simulink model "Sim_Ex25"  (R2017a)
settings: Solver=ode45  StartTime=0  StopTime=Stop_Time  MaxStep=Ts  RelTol=1e-3  EnableMultiTasking=on
values from neighbouring files (symbols this model uses):
  Lamf = 0.254    [A_Ex25.m]
  Lamf_Hat = 1.0*Lamf    (= 0.254)    [A_Ex25.m]
  Lds = 3.6e-3    (= 0.0036)    [A_Ex25.m]
  Lds_Hat = 1.0*Lds    (= 0.0036)    [A_Ex25.m]
  Lqs = 4.3e-3    (= 0.0043)    [A_Ex25.m]
  Lqs_Hat = 1.0*Lqs    (= 0.0043)    [A_Ex25.m]
  p = 3    [A_Ex25.m]
  Rs = 0.15    [A_Ex25.m]
  Step_Time = 0.05    [A_Ex25.m]
  Stop_Time = 0.25    [A_Ex25.m]
  Te_Rated = interp1(MTPA.Is(Ind_PosTe),MTPA.Te(Ind_PosTe),Is_Rated)    [A_Ex25.m]
  Te_Ref_Set = [0 1]*Te_Rated    [A_Ex25.m]
  Te_SlewRate = 10    [A_Ex25.m]
  Thetarm_Init = 0*pi*1/p    (= 0)    [A_Ex25.m]
  Ts = 1/fs    (= 5e-05)    [A_Ex25.m]
  Tsw = 1/fsw    (= 0.0001)    [A_Ex25.m]
  Vdc = 310    [A_Ex25.m]
  Wrm_Fin = 2000*2*pi/60    (= 209.439510239)    [A_Ex25.m]
  Wrm_Init = 2000*2*pi/60    (= 209.439510239)    [A_Ex25.m]
undefined symbols (not defined in the file or in its folder): CC, DiscIntNeverNeededParam, FW, Mode, MTPA
libraries: simulink x7
settings Model: SimulationMode=accelerator  Creator=KYC  LastModifiedBy=KYC
settings DataIOCC: LimitDataPoints=on  SaveFormat=Array
settings OptimizationCC: LifeSpan=inf
settings DebuggingCC: UnderspecifiedInitializationDetection=Classic  MergeDetectMultiDrivingBlocksExec=none  SolverPrmCheckMsg=warning  InheritedTsInSrcMsg=none  AllowSymbolicDim=off  StateNameClashWarn=warning  SFUnexpectedBacktrackingDiag=warning  SFNoUnconditionalDefaultTransitionDiag=warning  SFExecutionAtInitializationDiag=none
settings HardwareCC: ProdBitPerPointer=32  ProdBitPerSizeT=32  ProdBitPerPtrDiffT=32  ProdLargestAtomicFloat=None  ProdIntDivRoundTo=Undefined  ProdEndianess=Unspecified  ProdWordSize=32  ProdHWDeviceType=32-bit Generic
settings ModelReferenceCC: PropagateSignalLabelsOutOfModel=off
settings GRTTargetCC: TargetLangStandard=C89/C90 (ANSI)  GeneratePreprocessorConditionals=Disable all
settings ConfigComp: CovMetricSettings=dw  CovHtmlReporting=on  CovSaveCumulativeToWorkspaceVar=on  CovSaveSingleToWorkspaceVar=on  CovExternalEMLEnable=off  CovSFcnEnable=off

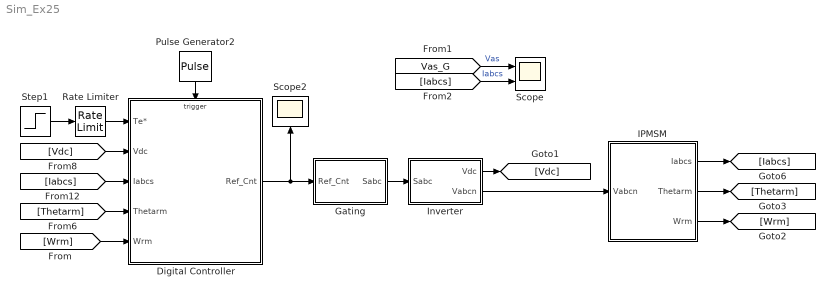
== system Sim_Ex25 ==
  Digital Controller : Subsystem
  Gating : Subsystem
  IPMSM : Subsystem
  Inverter : Subsystem
  Pulse Generator2 : DiscretePulseGenerator  PulseType=Time based  Period=Ts  PulseWidth=50
  Rate Limiter : RateLimiter  RisingSlewLimit=Te_SlewRate*Te_Rated  FallingSlewLimit=-Te_SlewRate*Te_Rated  SampleTimeMode=inherited
  Scope : Scope  NumInputPorts=2
  Scope2 : Scope
  Step1 : Step  Time=Step_Time  Before=Te_Ref_Set(:,1)  After=Te_Ref_Set(:,2)
  wires:
  Pulse Generator2/1 -> Digital Controller/Trigger
  [Vdc] -> Digital Controller/2(Vdc)
  Digital Controller/1(Ref_Cnt) -> Gating/1(Ref_Cnt), Scope2/1
  [Thetarm] -> Digital Controller/4(Thetarm)
  Gating/1(Sabc) -> Inverter/1(Sabc)
  [Iabcs] -> Digital Controller/3(Iabcs)
  Inverter/2(Vabcn) -> IPMSM/1(Vabcn)
  Inverter/1(Vdc) -> [Vdc]
  [Vas_G] -> Scope/1  "Vas"
  [Iabcs] -> Scope/2  "Iabcs"
  IPMSM/1(Iabcs) -> [Iabcs]
  IPMSM/2(Thetarm) -> [Thetarm]
  IPMSM/3(Wrm) -> [Wrm]
  Rate Limiter/1 -> Digital Controller/1(Te*)
  [Wrm] -> Digital Controller/5(Wrm)
  Step1/1 -> Rate Limiter/1

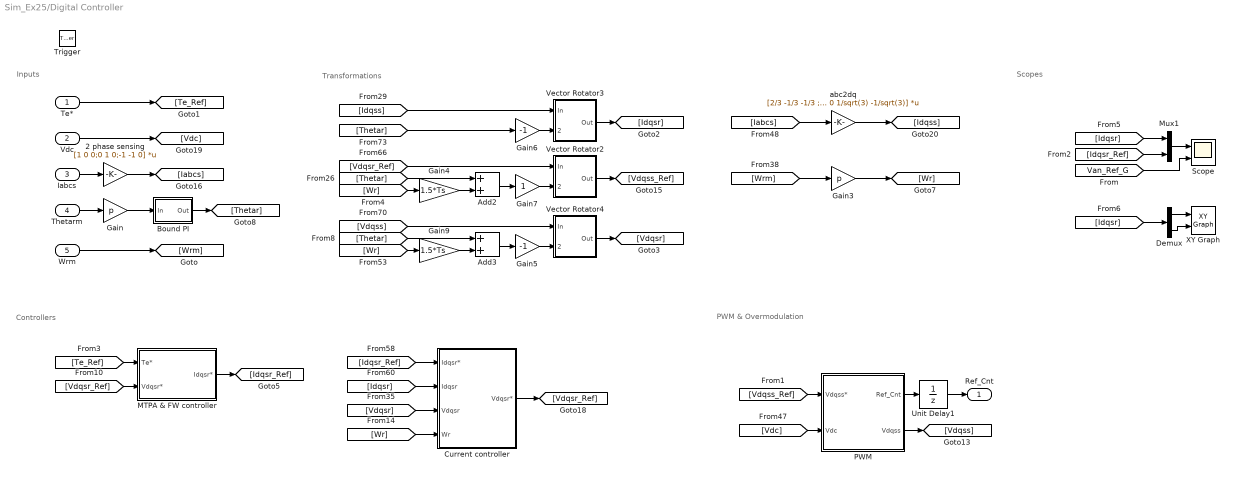
== system Sim_Ex25/Digital Controller ==
  note: PWM & Overmodulation
  note: Controllers
  note: Inputs
  note: Transformations
  note: Scopes
  Te* : Inport
  Vdc : Inport  Port=2
  Iabcs : Inport  Port=3
  Thetarm : Inport  Port=4
  Wrm : Inport  Port=5
  Trigger : TriggerPort  VariantControl=Variant
  2 phase sensing : Gain  Gain=[1 0 0;0 1 0;-1 -1 0]  Multiplication=Matrix(K*u)  SaturateOnIntegerOverflow=on  OutDataTypeStr=Inherit: Same as input  ParamDataTypeStr=Inherit: Same as input
  Add2 : Sum
  Add3 : Sum
  Bound PI : Subsystem
  Current controller : Subsystem
  Demux : Demux  Outputs=2
  Gain : Gain  Gain=p
  Gain3 : Gain  Gain=p
  Gain4 : Gain  Gain=1.5*Ts
  Gain5 : Gain  Gain=-1
  Gain6 : Gain  Gain=-1
  Gain7 : Gain
  Gain9 : Gain  Gain=1.5*Ts
  MTPA & FW controller : Subsystem
  Mux1 : Mux  Inputs=2
  PWM : Subsystem
  Scope : Scope  NumInputPorts=2
  Unit Delay1 : UnitDelay  SampleTime=-1
  Vector Rotator2 : Subsystem
  Vector Rotator3 : Subsystem
  Vector Rotator4 : Subsystem
  XY Graph : simulink/Sinks/XY Graph  xmin=-60  xmax=0  ymin=0  ymax=60  st=-1
  abc2dq : Gain  Gain=[2/3 -1/3 -1/3 ; 0 1/sqrt(3) -1/sqrt(3)]  Multiplication=Matrix(K*u)  SaturateOnIntegerOverflow=on  OutDataTypeStr=Inherit: Same as input  ParamDataTypeStr=Inherit: Same as input
  Ref_Cnt : Outport  InitialOutput=[0]
  wires:
  [Idqsr] -> Current controller/2(Idqsr)
  abc2dq/1 -> [Idqss]
  [Iabcs] -> abc2dq/1
  Vdc/1 -> [Vdc]
  [Vdqsr] -> Current controller/3(Vdqsr)
  [Idqsr_Ref] -> Current controller/1(Idqsr*)
  Thetarm/1 -> Gain/1
  [Wr] -> Current controller/4(Wr)
  Gain/1 -> Bound PI/1(In)
  Bound PI/1(Out) -> [Thetar]
  Current controller/1(Vdqsr*) -> [Vdqsr_Ref]
  Unit Delay1/1 -> Ref_Cnt/1
  PWM/2(Vdqss) -> [Vdqss]
  [Vdc] -> PWM/2(Vdc)
  Add2/1 -> Gain7/1
  Gain7/1 -> Vector Rotator2/2(Theta)
  [Vdqsr_Ref] -> Vector Rotator2/1(In)
  Vector Rotator2/1(Out) -> [Vdqss_Ref]
  [Wr] -> Gain9/1
  Gain9/1 -> Add3/2
  Add3/1 -> Gain5/1
  [Thetar] -> Add3/1
  Gain5/1 -> Vector Rotator4/2(Theta)
  [Vdqss] -> Vector Rotator4/1(In)
  Vector Rotator4/1(Out) -> [Vdqsr]
  [Vdqss_Ref] -> PWM/1(Vdqss*)
  Gain6/1 -> Vector Rotator3/2(Theta)
  [Idqss] -> Vector Rotator3/1(In)
  Vector Rotator3/1(Out) -> [Idqsr]
  [Thetar] -> Gain6/1
  PWM/1(Ref_Cnt) -> Unit Delay1/1
  Iabcs/1 -> 2 phase sensing/1
  2 phase sensing/1 -> [Iabcs]
  [Wr] -> Gain4/1
  Gain4/1 -> Add2/2
  [Thetar] -> Add2/1
  [Van_Ref_G] -> Scope/2
  Te*/1 -> [Te_Ref]
  [Idqsr] -> Demux/1
  Demux/2 -> XY Graph/2
  Demux/1 -> XY Graph/1
  [Idqsr_Ref] -> Mux1/2
  Mux1/1 -> Scope/1
  [Idqsr] -> Mux1/1
  [Vdqsr_Ref] -> MTPA & FW controller/2(Vdqsr*)
  MTPA & FW controller/1(Idqsr*) -> [Idqsr_Ref]
  [Te_Ref] -> MTPA & FW controller/1(Te*)
  [Wrm] -> Gain3/1
  Gain3/1 -> [Wr]
  Wrm/1 -> [Wrm]

== system Sim_Ex25/Gating ==
  Ref_Cnt : Inport
  Add3 : Sum  Inputs=+-
  Relay3 : Relay  OnSwitchValue=10*eps  OffSwitchValue=-10*eps  OutDataTypeStr=double
  Repeating Sequence1 : simulink/Sources/Repeating Sequence  rep_seq_t=[0 Tsw/2 Tsw]  rep_seq_y=[0 1 0]
  Sabc : Outport
  wires:
  Add3/1 -> Relay3/1
  Relay3/1 -> Sabc/1
  Repeating Sequence1/1 -> Add3/2
  Ref_Cnt/1 -> Add3/1

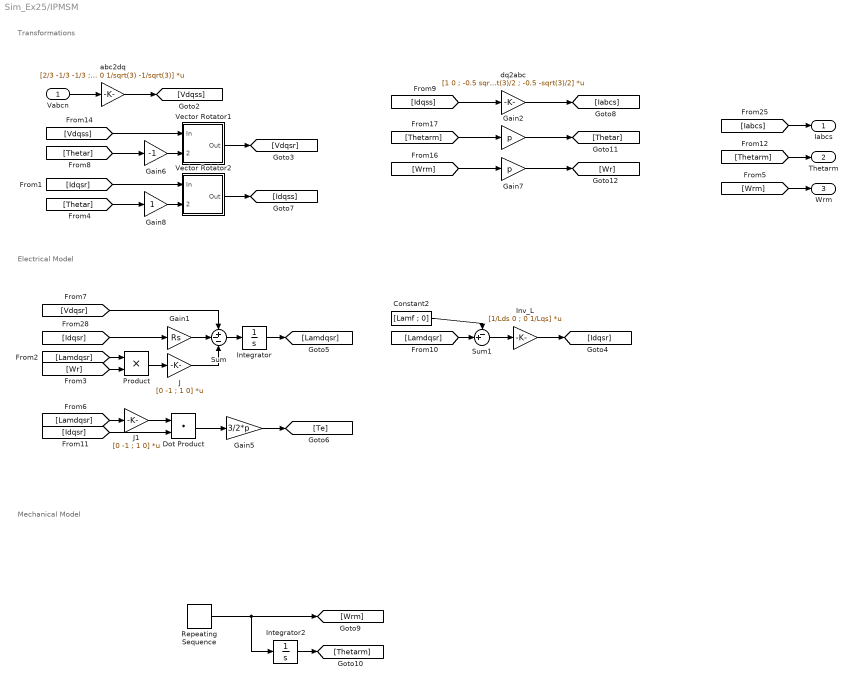
== system Sim_Ex25/IPMSM ==
  note: Transformations
  note: Electrical Model
  note: Mechanical Model
  Vabcn : Inport
  Constant2 : Constant  Value=[Lamf ; 0]
  Dot Product : DotProduct  InputSameDT=on  OutDataTypeStr=Inherit: Inherit via internal rule
  Gain1 : Gain  Gain=Rs
  Gain2 : Gain  Gain=p
  Gain5 : Gain  Gain=3/2*p
  Gain6 : Gain  Gain=-1
  Gain7 : Gain  Gain=p
  Gain8 : Gain
  Integrator : Integrator  InitialCondition=[Lamf ; 0]
  Integrator2 : Integrator  InitialCondition=Thetarm_Init  WrapState=on
  Inv_L : Gain  Gain=[1/Lds 0 ; 0 1/Lqs]  Multiplication=Matrix(K*u)
  J : Gain  Gain=[0 -1 ; 1 0]  Multiplication=Matrix(K*u)
  J1 : Gain  Gain=[0 -1 ; 1 0]  Multiplication=Matrix(K*u)
  Product : Product  RndMeth=Zero
  Repeating Sequence : simulink/Sources/Repeating Sequence  rep_seq_t=[0 Stop_Time]  rep_seq_y=[Wrm_Init Wrm_Fin]
  Sum : Sum  Inputs=+--
  Sum1 : Sum  Inputs=-+|
  Vector Rotator1 : Subsystem
  Vector Rotator2 : Subsystem
  abc2dq : Gain  Gain=[2/3 -1/3 -1/3 ; 0 1/sqrt(3) -1/sqrt(3)]  Multiplication=Matrix(K*u)  SaturateOnIntegerOverflow=on  OutDataTypeStr=Inherit: Same as input  ParamDataTypeStr=Inherit: Same as input
  dq2abc : Gain  Gain=[1 0 ; -0.5 sqrt(3)/2 ; -0.5 -sqrt(3)/2]  Multiplication=Matrix(K*u)
  Iabcs : Outport
  Thetarm : Outport  Port=2
  Wrm : Outport  Port=3
  wires:
  [Iabcs] -> Iabcs/1
  [Wrm] -> Gain7/1
  [Thetarm] -> Gain2/1
  Gain7/1 -> [Wr]
  dq2abc/1 -> [Iabcs]
  [Idqss] -> dq2abc/1
  Vector Rotator2/1(Out) -> [Idqss]
  [Idqsr] -> Vector Rotator2/1(In)
  Vector Rotator1/1(Out) -> [Vdqsr]
  [Thetarm] -> Thetarm/1
  Gain2/1 -> [Thetar]
  [Thetar] -> Gain6/1
  Gain6/1 -> Vector Rotator1/2(Theta)
  [Thetar] -> Gain8/1
  Gain8/1 -> Vector Rotator2/2(Theta)
  Integrator2/1 -> [Thetarm]
  Repeating Sequence/1 -> [Wrm], Integrator2/1
  Sum1/1 -> Inv_L/1
  Inv_L/1 -> [Idqsr]
  [Lamdqsr] -> Sum1/2
  Constant2/1 -> Sum1/1
  Dot Product/1 -> Gain5/1
  J1/1 -> Dot Product/1
  [Lamdqsr] -> J1/1
  [Idqsr] -> Dot Product/2
  Gain5/1 -> [Te]
  Integrator/1 -> [Lamdqsr]
  [Vdqsr] -> Sum/1
  [Lamdqsr] -> Product/1
  Sum/1 -> Integrator/1
  [Wr] -> Product/2
  Product/1 -> J/1
  [Idqsr] -> Gain1/1
  J/1 -> Sum/3
  Gain1/1 -> Sum/2
  Vabcn/1 -> abc2dq/1
  abc2dq/1 -> [Vdqss]
  [Vdqss] -> Vector Rotator1/1(In)
  [Wrm] -> Wrm/1

== system Sim_Ex25/Inverter ==
  Sabc : Inport
  Constant2 : Constant  Value=Vdc
  Gain : Gain  Gain=[1 0 0]  Multiplication=Matrix(K*u)
  Product1 : Product  RndMeth=Zero
  Relay2 : Relay  OnSwitchValue=0.5  OffSwitchValue=0.5  OnOutputValue=1/2  OffOutputValue=-1/2  OutDataTypeStr=double
  abcn to abcs : Subsystem
  Vdc : Outport
  Vabcn : Outport  Port=2
  tag scope: Vas_G=global
  wires:
  Constant2/1 -> Vdc/1, Product1/1
  Sabc/1 -> Relay2/1
  Relay2/1 -> Product1/2
  Product1/1 -> abcn to abcs/1(fabcn), Vabcn/1
  Gain/1 -> [Vas_G]
  abcn to abcs/1(fabcs) -> Gain/1

== system Sim_Ex25/Digital Controller/Bound PI ==
  In : Inport
  Fcn1 : Fcn  Expr=1/(2*pi)*u+0.5
  Fcn2 : Fcn  Expr=u-floor(u)
  Fcn3 : Fcn  Expr=2*pi*(u-0.5)
  Out : Outport
  wires:
  Fcn1/1 -> Fcn2/1
  Fcn2/1 -> Fcn3/1
  In/1 -> Fcn1/1
  Fcn3/1 -> Out/1

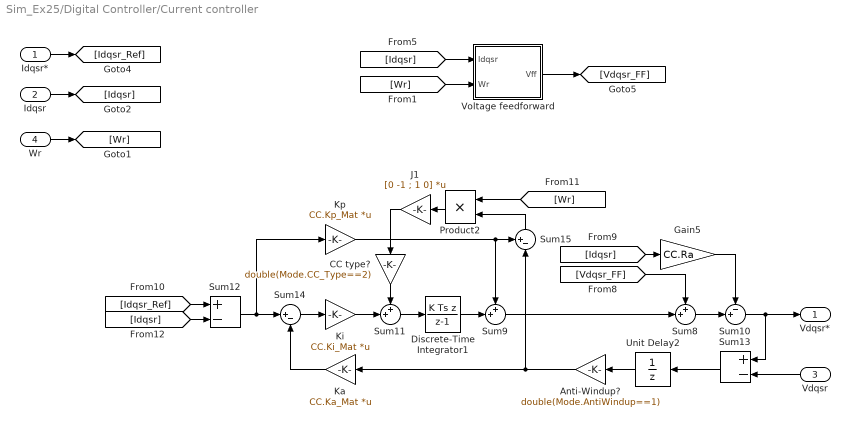
== system Sim_Ex25/Digital Controller/Current controller ==
  Idqsr* : Inport
  Idqsr : Inport  Port=2
  Vdqsr : Inport  Port=3
  Wr : Inport  Port=4
  Anti-Windup? : Gain  Gain=double(Mode.AntiWindup==1)
  CC type? : Gain  Gain=double(Mode.CC_Type==2)
  Discrete-Time Integrator1 : DiscreteIntegrator  IntegratorMethod=Integration: Backward Euler  SampleTime=-1  ICPrevOutput=DiscIntNeverNeededParam  ICPrevScaledInput=DiscIntNeverNeededParam
  Gain5 : Gain  Gain=CC.Ra
  J1 : Gain  Gain=[0 -1 ; 1 0]  Multiplication=Matrix(K*u)
  Ka : Gain  Gain=CC.Ka_Mat  Multiplication=Matrix(K*u)  SaturateOnIntegerOverflow=on  OutDataTypeStr=Inherit: Same as input  ParamDataTypeStr=Inherit: Same as input
  Ki : Gain  Gain=CC.Ki_Mat  Multiplication=Matrix(K*u)  SaturateOnIntegerOverflow=on  OutDataTypeStr=Inherit: Same as input  ParamDataTypeStr=Inherit: Same as input
  Kp : Gain  Gain=CC.Kp_Mat  Multiplication=Matrix(K*u)  SaturateOnIntegerOverflow=on  OutDataTypeStr=Inherit: Same as input  ParamDataTypeStr=Inherit: Same as input
  Product2 : Product  RndMeth=Zero
  Sum10 : Sum  Inputs=-+|
  Sum11 : Sum  Inputs=++|
  Sum12 : Sum  Inputs=+-
  Sum13 : Sum  Inputs=+-
  Sum14 : Sum  Inputs=|+-
  Sum15 : Sum  Inputs=+-|
  Sum8 : Sum  Inputs=++|
  Sum9 : Sum  Inputs=++|
  Unit Delay2 : UnitDelay  SampleTime=-1
  Voltage feedforward : Subsystem
  Vdqsr* : Outport
  wires:
  Idqsr/1 -> [Idqsr]
  Idqsr*/1 -> [Idqsr_Ref]
  Wr/1 -> [Wr]
  [Idqsr] -> Voltage feedforward/1(Idqsr)
  [Wr] -> Voltage feedforward/2(Wr)
  Voltage feedforward/1(Vff) -> [Vdqsr_FF]
  Discrete-Time Integrator1/1 -> Sum9/2
  Gain5/1 -> Sum10/1
  [Idqsr_Ref] -> Sum12/1
  Sum11/1 -> Discrete-Time Integrator1/1
  Ki/1 -> Sum11/2
  Kp/1 -> Sum15/1, Sum9/1
  Sum8/1 -> Sum10/2
  CC type?/1 -> Sum11/1
  [Idqsr] -> Gain5/1
  J1/1 -> CC type?/1
  Product2/1 -> J1/1
  Sum12/1 -> Sum14/1, Kp/1
  [Idqsr] -> Sum12/2
  Sum9/1 -> Sum8/2
  [Wr] -> Product2/1
  [Vdqsr_FF] -> Sum8/1
  Sum10/1 -> Vdqsr*/1, Sum13/1
  Vdqsr/1 -> Sum13/2
  Unit Delay2/1 -> Anti-Windup?/1
  Sum13/1 -> Unit Delay2/1
  Sum14/1 -> Ki/1
  Ka/1 -> Sum14/2
  Anti-Windup?/1 -> Sum15/2, Ka/1
  Sum15/1 -> Product2/2

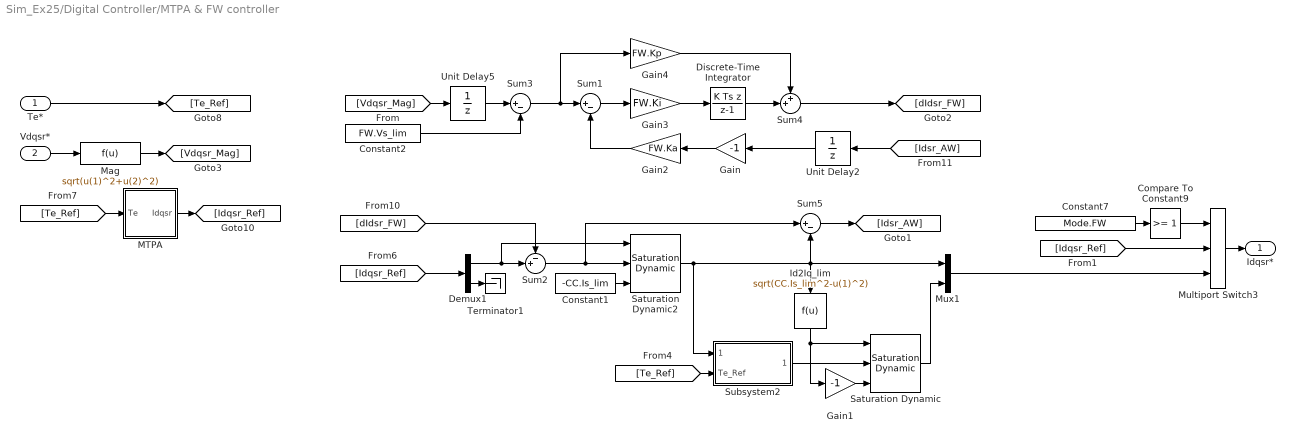
== system Sim_Ex25/Digital Controller/MTPA & FW controller ==
  Te* : Inport
  Vdqsr* : Inport  Port=2
  Compare To Constant9 : simulink/Logic and Bit Operations/Compare To Constant  relop=>=  const=1  OutDataTypeStr=boolean
  Constant1 : Constant  Value=-CC.Is_lim
  Constant2 : Constant  Value=FW.Vs_lim
  Constant7 : Constant  Value=Mode.FW
  Demux1 : Demux  Outputs=2
  Discrete-Time Integrator : DiscreteIntegrator  IntegratorMethod=Integration: Backward Euler  SampleTime=-1  ICPrevOutput=DiscIntNeverNeededParam  ICPrevScaledInput=DiscIntNeverNeededParam
  Gain : Gain  Gain=-1
  Gain1 : Gain  Gain=-1
  Gain2 : Gain  Gain=FW.Ka
  Gain3 : Gain  Gain=FW.Ki
  Gain4 : Gain  Gain=FW.Kp
  Id2Iq_lim : Fcn  Expr=sqrt(CC.Is_lim^2-u(1)^2)
  MTPA : Subsystem
  Mag : Fcn  Expr=sqrt(u(1)^2+u(2)^2)
  Multiport Switch3 : MultiPortSwitch  DataPortOrder=Zero-based contiguous  Inputs=2  OutDataTypeStr=double
  Mux1 : Mux  Inputs=[1 1]
  Saturation Dynamic : simulink/Discontinuities/Saturation Dynamic  OutMin=[]  OutMax=[]  OutDataTypeStr=Inherit: Same as second input  OutDataType=fixdt(1, 16)  OutScaling=2^-10  DoSatur=off
  Saturation Dynamic2 : simulink/Discontinuities/Saturation Dynamic  OutMin=[]  OutMax=[]  OutDataTypeStr=Inherit: Same as second input  OutDataType=fixdt(1, 16)  OutScaling=2^-10  DoSatur=off
  Subsystem2 : Subsystem
  Sum1 : Sum  Inputs=|+-
  Sum2 : Sum  Inputs=-+|
  Sum3 : Sum  Inputs=|+-
  Sum4 : Sum  Inputs=++|
  Sum5 : Sum  Inputs=|+-
  Terminator1 : Terminator
  Unit Delay2 : UnitDelay  SampleTime=-1
  Unit Delay5 : UnitDelay  SampleTime=-1
  Idqsr* : Outport
  wires:
  Demux1/1 -> Saturation Dynamic2/1, Sum2/2
  Saturation Dynamic2/1 -> Subsystem2/1(Idsr_Ref), Sum5/2, Id2Iq_lim/1, Mux1/1
  Saturation Dynamic/1 -> Mux1/2
  Id2Iq_lim/1 -> Saturation Dynamic/1, Gain1/1
  Gain1/1 -> Saturation Dynamic/3
  Sum2/1 -> Saturation Dynamic2/2, Sum5/1
  [Idqsr_Ref] -> Demux1/1
  Te*/1 -> [Te_Ref]
  [Te_Ref] -> MTPA/1(Te)
  MTPA/1(Idqsr) -> [Idqsr_Ref]
  [Te_Ref] -> Subsystem2/2(Te_Ref)
  Constant1/1 -> Saturation Dynamic2/3
  [dIdsr_FW] -> Sum2/1
  Sum5/1 -> [Idsr_AW]
  Subsystem2/1(Iqsr_Ref) -> Saturation Dynamic/2
  Constant7/1 -> Compare To Constant9/1
  Compare To Constant9/1 -> Multiport Switch3/1
  Multiport Switch3/1 -> Idqsr*/1
  [Idqsr_Ref] -> Multiport Switch3/2
  Mux1/1 -> Multiport Switch3/3
  Demux1/2 -> Terminator1/1
  Sum4/1 -> [dIdsr_FW]
  Gain2/1 -> Sum1/2
  Unit Delay2/1 -> Gain/1
  Vdqsr*/1 -> Mag/1
  Constant2/1 -> Sum3/2
  Gain4/1 -> Sum4/1
  Discrete-Time Integrator/1 -> Sum4/2
  Sum1/1 -> Gain3/1
  Gain3/1 -> Discrete-Time Integrator/1
  Sum3/1 -> Gain4/1, Sum1/1
  [Idsr_AW] -> Unit Delay2/1
  Gain/1 -> Gain2/1
  Mag/1 -> [Vdqsr_Mag]
  [Vdqsr_Mag] -> Unit Delay5/1
  Unit Delay5/1 -> Sum3/1

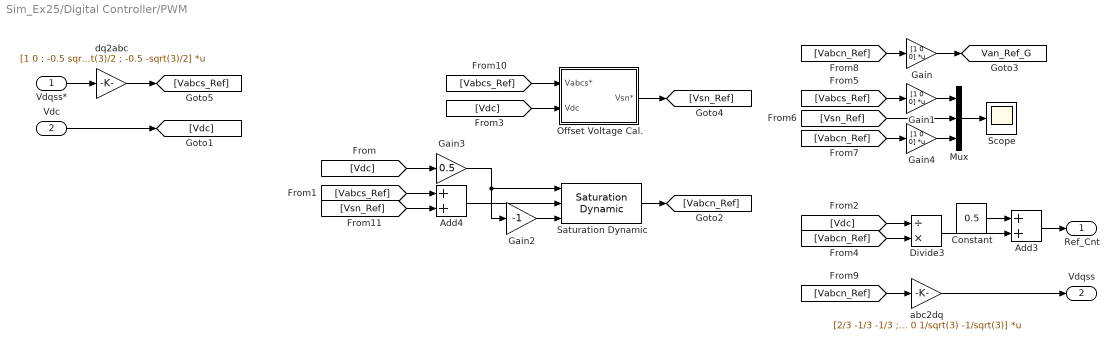
== system Sim_Ex25/Digital Controller/PWM ==
  Vdqss* : Inport
  Vdc : Inport  Port=2
  Add3 : Sum
  Add4 : Sum
  Constant : Constant  Value=0.5
  Divide3 : Product  Inputs=/*
  Gain : Gain  Gain=[1 0 0]  Multiplication=Matrix(K*u)
  Gain1 : Gain  Gain=[1 0 0]  Multiplication=Matrix(K*u)
  Gain2 : Gain  Gain=-1
  Gain3 : Gain  Gain=0.5
  Gain4 : Gain  Gain=[1 0 0]  Multiplication=Matrix(K*u)
  Mux : Mux  Inputs=3
  Offset Voltage Cal. : Subsystem
  Saturation Dynamic : simulink/Discontinuities/Saturation Dynamic  OutMin=[]  OutMax=[]  OutDataTypeStr=Inherit: Same as second input  OutDataType=fixdt(1, 16)  OutScaling=2^-10  DoSatur=off
  Scope : Scope
  abc2dq : Gain  Gain=[2/3 -1/3 -1/3 ; 0 1/sqrt(3) -1/sqrt(3)]  Multiplication=Matrix(K*u)  SaturateOnIntegerOverflow=on  OutDataTypeStr=Inherit: Same as input  ParamDataTypeStr=Inherit: Same as input
  dq2abc : Gain  Gain=[1 0 ; -0.5 sqrt(3)/2 ; -0.5 -sqrt(3)/2]  Multiplication=Matrix(K*u)
  Ref_Cnt : Outport
  Vdqss : Outport  Port=2
  tag scope: Van_Ref_G=global
  wires:
  Vdqss*/1 -> dq2abc/1
  dq2abc/1 -> [Vabcs_Ref]
  [Vabcs_Ref] -> Add4/1
  [Vsn_Ref] -> Add4/2
  Gain3/1 -> Saturation Dynamic/1, Gain2/1
  Gain2/1 -> Saturation Dynamic/3
  Add4/1 -> Saturation Dynamic/2
  Vdc/1 -> [Vdc]
  [Vdc] -> Gain3/1
  Mux/1 -> Scope/1
  [Vabcs_Ref] -> Gain1/1
  Gain1/1 -> Mux/1
  [Vsn_Ref] -> Mux/2
  Gain4/1 -> Mux/3
  [Vabcn_Ref] -> Gain4/1
  Saturation Dynamic/1 -> [Vabcn_Ref]
  abc2dq/1 -> Vdqss/1
  [Vabcn_Ref] -> abc2dq/1
  [Vabcs_Ref] -> Offset Voltage Cal./1(Vabcs*)
  [Vdc] -> Offset Voltage Cal./2(Vdc)
  Offset Voltage Cal./1(Vsn*) -> [Vsn_Ref]
  Divide3/1 -> Add3/2
  [Vabcn_Ref] -> Divide3/2
  Constant/1 -> Add3/1
  Add3/1 -> Ref_Cnt/1
  [Vdc] -> Divide3/1
  [Vabcn_Ref] -> Gain/1
  Gain/1 -> [Van_Ref_G]

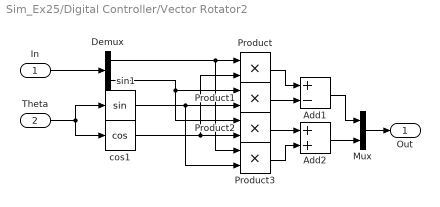
== system Sim_Ex25/Digital Controller/Vector Rotator2 ==
  In : Inport
  Theta : Inport  Port=2
  Add1 : Sum  Inputs=+-
  Add2 : Sum
  Demux : Demux  Outputs=2
  Mux : Mux  Inputs=[1 1]
  Product{,1..3} (4 alike) : Product  RndMeth=Zero
  cos1 : Trigonometry  Operator=cos
  sin1 : Trigonometry
  Out : Outport
  wires:
  Theta/1 -> cos1/1, sin1/1
  Demux/1 -> Product3/1, Product/1
  Mux/1 -> Out/1
  In/1 -> Demux/1
  Demux/2 -> Product1/1, Product2/1
  cos1/1 -> Product/2, Product2/2
  sin1/1 -> Product1/2, Product3/2
  Product/1 -> Add1/1
  Product1/1 -> Add1/2
  Add1/1 -> Mux/1
  Product2/1 -> Add2/1
  Product3/1 -> Add2/2
  Add2/1 -> Mux/2

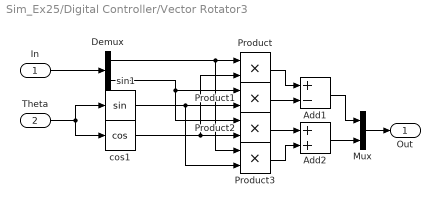
== system Sim_Ex25/Digital Controller/Vector Rotator3 ==
  In : Inport
  Theta : Inport  Port=2
  Add1 : Sum  Inputs=+-
  Add2 : Sum
  Demux : Demux  Outputs=2
  Mux : Mux  Inputs=[1 1]
  Product{,1..3} (4 alike) : Product  RndMeth=Zero
  cos1 : Trigonometry  Operator=cos
  sin1 : Trigonometry
  Out : Outport
  wires:
  Theta/1 -> cos1/1, sin1/1
  Demux/1 -> Product3/1, Product/1
  Mux/1 -> Out/1
  In/1 -> Demux/1
  Demux/2 -> Product1/1, Product2/1
  cos1/1 -> Product/2, Product2/2
  sin1/1 -> Product1/2, Product3/2
  Product/1 -> Add1/1
  Product1/1 -> Add1/2
  Add1/1 -> Mux/1
  Product2/1 -> Add2/1
  Product3/1 -> Add2/2
  Add2/1 -> Mux/2

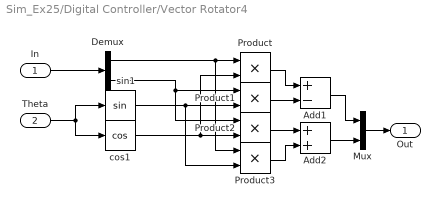
== system Sim_Ex25/Digital Controller/Vector Rotator4 ==
  In : Inport
  Theta : Inport  Port=2
  Add1 : Sum  Inputs=+-
  Add2 : Sum
  Demux : Demux  Outputs=2
  Mux : Mux  Inputs=[1 1]
  Product{,1..3} (4 alike) : Product  RndMeth=Zero
  cos1 : Trigonometry  Operator=cos
  sin1 : Trigonometry
  Out : Outport
  wires:
  Add2/1 -> Mux/2
  Product3/1 -> Add2/2
  Product2/1 -> Add2/1
  Add1/1 -> Mux/1
  Product1/1 -> Add1/2
  Product/1 -> Add1/1
  sin1/1 -> Product3/2, Product1/2
  cos1/1 -> Product2/2, Product/2
  Demux/2 -> Product2/1, Product1/1
  In/1 -> Demux/1
  Mux/1 -> Out/1
  Demux/1 -> Product/1, Product3/1
  Theta/1 -> sin1/1, cos1/1

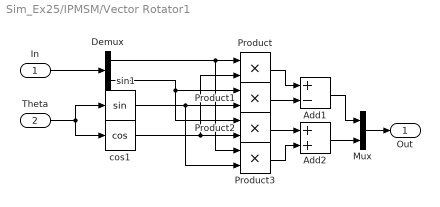
== system Sim_Ex25/IPMSM/Vector Rotator1 ==
  In : Inport
  Theta : Inport  Port=2
  Add1 : Sum  Inputs=+-
  Add2 : Sum
  Demux : Demux  Outputs=2
  Mux : Mux  Inputs=[1 1]
  Product{,1..3} (4 alike) : Product  RndMeth=Zero
  cos1 : Trigonometry  Operator=cos
  sin1 : Trigonometry
  Out : Outport
  wires:
  Add2/1 -> Mux/2
  Product3/1 -> Add2/2
  Product2/1 -> Add2/1
  Add1/1 -> Mux/1
  Product1/1 -> Add1/2
  Product/1 -> Add1/1
  sin1/1 -> Product3/2, Product1/2
  cos1/1 -> Product2/2, Product/2
  Demux/2 -> Product2/1, Product1/1
  In/1 -> Demux/1
  Mux/1 -> Out/1
  Demux/1 -> Product/1, Product3/1
  Theta/1 -> sin1/1, cos1/1

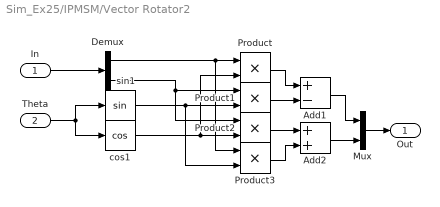
== system Sim_Ex25/IPMSM/Vector Rotator2 ==
  In : Inport
  Theta : Inport  Port=2
  Add1 : Sum  Inputs=+-
  Add2 : Sum
  Demux : Demux  Outputs=2
  Mux : Mux  Inputs=[1 1]
  Product{,1..3} (4 alike) : Product  RndMeth=Zero
  cos1 : Trigonometry  Operator=cos
  sin1 : Trigonometry
  Out : Outport
  wires:
  Theta/1 -> cos1/1, sin1/1
  Demux/1 -> Product3/1, Product/1
  Mux/1 -> Out/1
  In/1 -> Demux/1
  Demux/2 -> Product1/1, Product2/1
  cos1/1 -> Product/2, Product2/2
  sin1/1 -> Product1/2, Product3/2
  Product/1 -> Add1/1
  Product1/1 -> Add1/2
  Add1/1 -> Mux/1
  Product2/1 -> Add2/1
  Product3/1 -> Add2/2
  Add2/1 -> Mux/2

== system Sim_Ex25/Inverter/abcn to abcs ==
  fabcn : Inport
  Add1 : Sum  Inputs=+-
  Gain2 : Gain  Gain=1/3
  Sum of Elements : Sum  Inputs=+
  fabcs : Outport
  wires:
  Gain2/1 -> Add1/2
  Add1/1 -> fabcs/1
  Sum of Elements/1 -> Gain2/1
  fabcn/1 -> Add1/1, Sum of Elements/1

== system Sim_Ex25/Digital Controller/Current controller/Voltage feedforward ==
  Idqsr : Inport
  Wr : Inport  Port=2
  CC type : Gain  Gain=double(Mode.CC_Type==1)
  Constant : Constant  Value=[Lamf_Hat;0]
  J : Gain  Gain=[0 -1 ; 1 0]  Multiplication=Matrix(K*u)
  L_Hat : Gain  Gain=[Lds_Hat 0 ; 0 Lqs_Hat]  Multiplication=Matrix(K*u)
  Product : Product  RndMeth=Zero
  Sum2 : Sum  Inputs=|++
  Vff : Outport
  wires:
  Idqsr/1 -> L_Hat/1
  Wr/1 -> Product/2
  J/1 -> Product/1
  Product/1 -> Vff/1
  L_Hat/1 -> CC type/1
  Sum2/1 -> J/1
  CC type/1 -> Sum2/1
  Constant/1 -> Sum2/2

== system Sim_Ex25/Digital Controller/MTPA & FW controller/MTPA ==
  Te : Inport
  1-D Lookup Table : Lookup_n-D  NumberOfTableDimensions=1  BreakpointsForDimension1=MTPA.Te  Table=MTPA.Iqsr  InternalRulePriority=Speed  RndMeth=Simplest  InputSameDT=on
  1-D Lookup Table1 : Lookup_n-D  NumberOfTableDimensions=1  BreakpointsForDimension1=MTPA.Te  Table=MTPA.Idsr  InternalRulePriority=Speed  RndMeth=Simplest  InputSameDT=on
  Mux : Mux  Inputs=2
  Idqsr : Outport
  wires:
  Te/1 -> 1-D Lookup Table1/1, 1-D Lookup Table/1
  Mux/1 -> Idqsr/1
  1-D Lookup Table1/1 -> Mux/1
  1-D Lookup Table/1 -> Mux/2

== system Sim_Ex25/Digital Controller/MTPA & FW controller/Subsystem2 ==
  Idsr_Ref : Inport
  Te_Ref : Inport  Port=2
  Add1 : Sum
  Constant : Constant  Value=Lamf_Hat
  Divide : Product  Inputs=*/
  Gain2 : Gain  Gain=2/3/p
  Gain5 : Gain  Gain=Lds_Hat-Lqs_Hat
  Iqsr_Ref : Outport
  wires:
  Gain5/1 -> Add1/1
  Te_Ref/1 -> Gain2/1
  Constant/1 -> Add1/2
  Gain2/1 -> Divide/1
  Add1/1 -> Divide/2
  Idsr_Ref/1 -> Gain5/1
  Divide/1 -> Iqsr_Ref/1

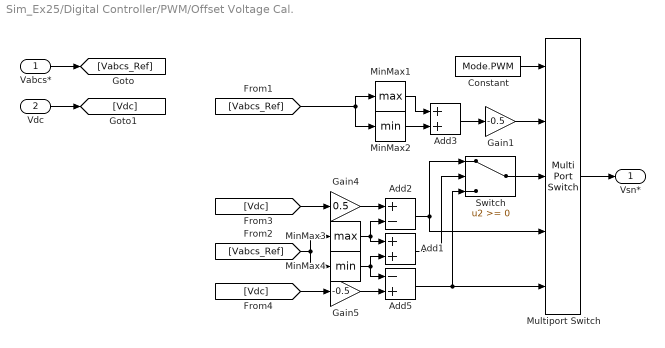
== system Sim_Ex25/Digital Controller/PWM/Offset Voltage Cal. ==
  Vabcs* : Inport
  Vdc : Inport  Port=2
  Add1 : Sum
  Add2 : Sum  Inputs=+-
  Add3 : Sum
  Add5 : Sum  Inputs=-+
  Constant : Constant  Value=Mode.PWM
  Gain1 : Gain  Gain=-0.5
  Gain4 : Gain  Gain=0.5
  Gain5 : Gain  Gain=-0.5
  MinMax1 : MinMax  Function=max
  MinMax2 : MinMax
  MinMax3 : MinMax  Function=max
  MinMax4 : MinMax
  Multiport Switch : MultiPortSwitch  Inputs=4
  Switch : Switch
  Vsn* : Outport
  wires:
  Add2/1 -> Multiport Switch/4, Switch/1
  Add3/1 -> Gain1/1
  MinMax2/1 -> Add3/2
  MinMax1/1 -> Add3/1
  Constant/1 -> Multiport Switch/1
  Gain1/1 -> Multiport Switch/2
  MinMax3/1 -> Add2/2, Add1/1
  [Vabcs_Ref] -> MinMax3/1, MinMax4/1
  [Vabcs_Ref] -> MinMax2/1, MinMax1/1
  Multiport Switch/1 -> Vsn*/1
  Add1/1 -> Switch/2
  MinMax4/1 -> Add1/2, Add5/1
  Gain4/1 -> Add2/1
  Switch/1 -> Multiport Switch/3
  [Vdc] -> Gain5/1
  Gain5/1 -> Add5/2
  Add5/1 -> Switch/3, Multiport Switch/5
  [Vdc] -> Gain4/1
  Vabcs*/1 -> [Vabcs_Ref]
  Vdc/1 -> [Vdc]
